simulink model "ModerForM"  (R2013a)
settings: Solver=ode3  StartTime=0.0  StopTime=0.0050  FixedStep=1e-7  MaxStep=1e-6  RelTol=1e-3
libraries: simulink x1
settings Model: Creator=pankx  LastModifiedBy=pankx
settings DataIOCC: SignalLoggingSaveFormat=ModelDataLogs  InspectSignalLogs=on
settings OptimizationCC: InitFltsAndDblsToZero=on
settings DebuggingCC: SaveWithParameterizedLinksMsg=none  SignalResolutionControl=TryResolveAllWithWarning  MultiTaskDSMMsg=warning  MultiTaskCondExecSysMsg=none  FcnCallInpInsideContextMsg=UseLocalSettings  StrictBusMsg=Warning
settings RTWCC: IncludeERTFirstTime=on
settings GRTTargetCC: TargetFcnLib=ansi_tfl_tmw.mat  CombineOutputUpdateFcns=off  GRTInterface=on

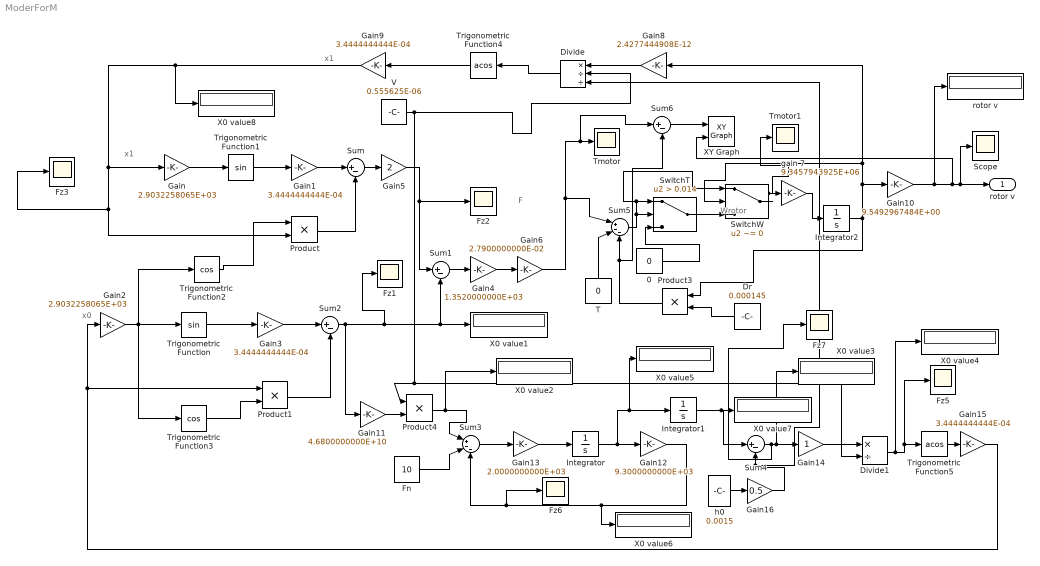
== system ModerForM ==
  note: x0
  note: x1
  note: F
  note: Wrotor
  note: x1
   X0 value{1..8} (8 alike) : Display
  0 : Constant  Value=0
  Divide : Product  Inputs=*//
  Divide1 : Product  Inputs=*/
  Dr : Constant  Value=0.000145
  Fn : Constant  Value=10
  Fz{1..3,5..7} (6 alike) : Scope
      Fz1 settings: TimeRange=0.0025  YMin=0.00286513  YMax=0.00316673  SaveName=ScopeData5  MaxDataPoints=50000
      Fz2 settings: TimeRange=0.0025  YMin=528.593  YMax=584.235  SaveName=ScopeData6  MaxDataPoints=50000
      Fz3 settings: TimeRange=0.0025  YMin=0.000379204  YMax=0.00037921  SaveName=ScopeData7  MaxDataPoints=50000
      Fz5 settings: TimeRange=0.0025  YMin=-1361.75  YMax=-1359  MaxDataPoints=50000
      Fz6 settings: TimeRange=0.0025  YMin=16.369  YMax=18.092  SaveName=ScopeData2  MaxDataPoints=50000
      Fz7 settings: TimeRange=0.0025  YMin=0.00099484  YMax=0.00109956  MaxDataPoints=50000
  Gain : Gain  Gain=2.9032258065E+03
  Gain{1,3,9,15} (4 alike) : Gain  Gain=3.4444444444E-04
  Gain10 : Gain  Gain=9.5492967484E+00
  Gain11 : Gain  Gain=4.6800000000E+10
  Gain12 : Gain  Gain=9.3000000000E+03
  Gain13 : Gain  Gain=2.0000000000E+03
  Gain14 : Gain
  Gain16 : Gain  Gain=0.5
  Gain2 : Gain  Gain=2.9032258065E+03
  Gain4 : Gain  Gain=1.3520000000E+03
  Gain5 : Gain  Gain=2
  Gain6 : Gain  Gain=2.7900000000E-02
  Gain8 : Gain  Gain=2.4277444908E-12
  Integrator : Integrator
  Integrator1 : Integrator  InitialCondition=0.00075
  Integrator2 : Integrator
  Product{,1,3..4} (4 alike) : Product  RndMeth=Zero
  Scope : Scope
      settings: TimeRange=0.0025  YMin=724  YMax=729.75  SaveName=WD4  MaxDataPoints=20000
  Sum{,1..2,4,6} (5 alike) : Sum  Inputs=|+-
  Sum3 : Sum  Inputs=|+--
  Sum5 : Sum  Inputs=|+--
  SwitchT : Switch  Criteria=u2 > Threshold  Threshold=0.014
  SwitchW : Switch  Criteria=u2 ~= 0
  T : Constant  Value=0
  Tmotor : Scope
      settings: TimeRange=0.0025  YMin=0.0144378  YMax=0.0144378  SaveName=TD4  MaxDataPoints=20000
  Tmotor1 : Scope
      settings: TimeRange=0.0025  YMin=0.01154  YMax=0.01169  SaveName=ToutD4  MaxDataPoints=20000
  Trigonometric Function : Trigonometry
  Trigonometric Function1 : Trigonometry
  Trigonometric Function2 : Trigonometry  Operator=cos
  Trigonometric Function3 : Trigonometry  Operator=cos
  Trigonometric Function4 : Trigonometry  Operator=acos
  Trigonometric Function5 : Trigonometry  Operator=acos
  V : Constant  Value=0.555625E-06
  XY Graph : simulink/Sinks/XY Graph  xmin=0  xmax=0.03  ymin=0  ymax=1000  st=-1
  gain 7 : Gain  Gain=9.3457943925E+06
  h0 : Constant  Value=0.0015
  rotor v : Display
  "rotor v " : Outport
  wires:
  Gain/1 -> Trigonometric Function1/1
  Trigonometric Function1/1 -> Gain1/1
  Gain1/1 -> Sum/1
  Sum/1 -> Gain5/1
  Trigonometric Function2/1 -> Product/1
  Gain5/1 -> Fz2/1, Sum1/1
  Trigonometric Function/1 -> Gain3/1
  Gain3/1 -> Sum2/1
  Trigonometric Function3/1 -> Product1/2
  Product1/1 -> Sum2/2
  Fn/1 -> Sum3/2
  Gain12/1 -> " X0 value6"/1, Fz6/1, Sum3/3
  Sum2/1 -> Fz1/1, " X0 value1"/1, Sum1/2, Gain11/1
  Gain2/1 -> Trigonometric Function2/1, Trigonometric Function3/1, Trigonometric Function/1
  Sum3/1 -> Gain13/1
  Gain13/1 -> Integrator/1
  Integrator/1 -> " X0 value5"/1, Integrator1/1, Gain12/1
  Trigonometric Function4/1 -> Gain9/1
  Product/1 -> Sum/2
  Sum1/1 -> Gain4/1
  Gain4/1 -> Gain6/1
  Sum5/1 -> SwitchW/1, SwitchT/1, SwitchT/2
  gain 7/1 -> Integrator2/1
  Gain10/1 -> rotor v/1, XY Graph/2, "rotor v "/1, Scope/1
  T/1 -> Sum5/2
  Trigonometric Function5/1 -> Gain15/1
  Integrator2/1 -> Product3/1, SwitchW/2, Gain8/1, Gain10/1
  Dr/1 -> Product3/2
  Product3/1 -> Sum6/2, Sum5/3
  Gain8/1 -> Divide/1
  Divide/1 -> Trigonometric Function4/1
  V/1 -> Divide/2, Product4/1, Divide1/2
  Gain11/1 -> Product4/2
  Product4/1 -> " X0 value2"/1, Sum3/1
  h0/1 -> Gain16/1
  Gain16/1 -> Sum4/2, Divide/3
  Sum4/1 -> Fz7/1, " X0 value3"/1, Gain14/1
  Gain14/1 -> Divide1/1
  Divide1/1 -> " X0 value4"/1, Fz5/1, Trigonometric Function5/1
  Integrator1/1 -> " X0 value7"/1, Sum4/1
  Gain9/1 -> " X0 value8"/1, Fz3/1, Product/2, Gain/1
  0/1 -> SwitchT/3
  SwitchT/1 -> SwitchW/3
  Gain15/1 -> Product1/1, Gain2/1
  Gain6/1 -> Sum5/1, Sum6/1, Tmotor/1
  SwitchW/1 -> gain 7/1, Tmotor1/1
  Sum6/1 -> XY Graph/1
